simulink model "regcontrol_model"  (Simulink 9.1)
settings: Solver=VariableStepAuto  StartTime=0.0  StopTime=10.0  RelTol=1e-3
values from neighbouring files (symbols this model uses):
  BandWidth = Simulink.Parameter    [start.m]
  BaseVoltage = Simulink.Parameter    [start.m]
  CogenEnabled = false    [regcontrol_emulator.m]    (also in start.m = Simulink.Parameter)
  IsReversible = Simulink.Parameter    [start.m]
  LDC_Z = Simulink.Parameter    [start.m]
  PTratio = Simulink.Parameter    [start.m]
  RevBand = Simulink.Parameter    [start.m]
  RevVreg = Simulink.Parameter    [start.m]
  TapLimitPerChange = Simulink.Parameter    [start.m]
  UsingRegulatedBus = Simulink.Parameter    [start.m]
  Vlimit = Simulink.Parameter    [start.m]
  Vreg = Simulink.Parameter    [start.m]
undefined symbols (not defined in the file or in its folder): ControlModes, m, n
libraries: simulink x3
(part 2 of 2)

== stateflow chart Queue Handler ==
  settings: enableNonTerminalStates=1
  state Executive [parallel]
    settings: executionOrder=1
    state Asleep
      ex: Status.data = Statuses.READY; % reset status
      INTERNAL_DONE = false;
      EXECUTIVE_DONE = false;
    state DoNearestActions
      state WaitOnPeek
        en: send(QUEUE_PEEK, Internal);
      state WaitOnPop
        en: send(QUEUE_POP, Internal);
      state ErrorNoItems
        en: Status.data = ...
        Statuses.ERROR;
        send(Status);
      (default) -> (junction 902) : % do only those actions with the same delay time as the first action time return time
          | {q_len_initial = GetQueueSize;
          | PendingActionsCompleted = false; % local for now
          | }
      (junction 902) -> (junction 903) [order 1] : [q_len_initial > 0]
      (junction 902) -> Executive.DoNearestActions.ErrorNoItems [order 2]
      (junction 903) -> WaitOnPeek : {INTERNAL_DONE = false;
          | ActionTime = ExternalAT; % peek with given AT
          | }
      (junction 905) -> (junction 904) [order 1] : [jj <= q_len_initial]
      (junction 904) -> Executive.DoNearestActions.WaitOnPop : {INTERNAL_DONE = false;}
      WaitOnPeek -> (junction 905) : [INTERNAL_DONE]
          | {ActionTime = Out(QF.Time);
          | QHour = Out(QF.Hour);
          | QSec = Out(QF.Sec);
          | jj = 1;}
      Executive.DoNearestActions.WaitOnPop -> (junction 906) : [INTERNAL_DONE]
          | %send(DoPendingAction);
      (junction 906) -> (junction 905) : {jj = jj + 1;}
      (junction 905) -> (junction 908) [order 2]
      Executive.DoNearestActions.ErrorNoItems -> (junction 907)
      (junction 908) -> (junction 907)
      (junction 907) -> (junction 909) : {EXECUTIVE_DONE = true;}
    state DoAllActions
      state WaitOnPop
        en: send(QUEUE_POP, Internal);
      state ErrorNoItems
        en: Status.data = ...
        Statuses.ERROR;
        send(Status);
      (default) -> (junction 923) : {q_len_initial = GetQueueSize;}
      (junction 923) -> (junction 924) [order 1] : [q_len_initial ~= 0]
      (junction 923) -> Executive.DoAllActions.ErrorNoItems [order 2]
      (junction 924) -> (junction 926) : {ActionTime = ExternalAT;
          | jj = 1;}
      (junction 926) -> (junction 925) [order 1] : [jj <= q_len_initial]
      (junction 925) -> Executive.DoAllActions.WaitOnPop : {INTERNAL_DONE = false;}
      (junction 927) -> (junction 926) : {jj = jj + 1;}
      (junction 926) -> (junction 929) [order 2]
      Executive.DoAllActions.WaitOnPop -> (junction 927) : [INTERNAL_DONE]
          | %send(DoPendingAction);
      Executive.DoAllActions.ErrorNoItems -> (junction 928)
      (junction 929) -> (junction 928)
      (junction 928) -> (junction 930) : {EXECUTIVE_DONE = true;}
    state Pushing
      en: send(QUEUE_PUSH, Internal);
    state DeletingByHandle
      en: send(QUEUE_DELETE, Internal);
    state Peeking
      en: send(QUEUE_PEEK, Internal);
    state Popping
      en: send(QUEUE_POP, Internal);
    state ReadyAgain
      Status.data = Statuses.READY;
      send(Status);
    Executive.Asleep -> Executive.DeletingByHandle [order 6] : QueueAction[QueueAction.data == ...
        | QueueActions.DELETE]
    Executive.Asleep -> Executive.Peeking [order 5] : QueueAction[QueueAction.data == ...
        | QueueActions.PEEK]
    Executive.Asleep -> Executive.Popping [order 4] : QueueAction[QueueAction.data == ...
        | QueueActions.POP]
    (default) -> Executive.Asleep
    Executive.Asleep -> Executive.Pushing [order 3] : QueueAction[QueueAction.data == ...
        | QueueActions.PUSH]
    Executive.Asleep -> DoAllActions [order 2] : QueueAction[QueueAction.data == ...
        | QueueActions.DO_ALL_ACTIONS]
    ReadyAgain -> Executive.Asleep
    Executive.Asleep -> DoNearestActions [order 1] : QueueAction[QueueAction.data == DO_NEAREST_ACTIONS]
    Executive.Pushing -> ReadyAgain : [INTERNAL_DONE]
    Executive.Popping -> ReadyAgain : [INTERNAL_DONE]
    Executive.DeletingByHandle -> ReadyAgain : [INTERNAL_DONE]
    Executive.Peeking -> ReadyAgain : [INTERNAL_DONE]
    DoAllActions -> ReadyAgain : [EXECUTIVE_DONE]
    DoNearestActions -> ReadyAgain : [EXECUTIVE_DONE]
  state Internal [parallel]
    settings: executionOrder=2
    state Asleep
    state Popping
      (default) -> (junction 955) : % delete from beginning, t<= ActionTime:
          | {q_len = GetQueueSize;
          | ii = 1;
          | }
      (junction 955) -> (junction 952) [order 1] : [ii <= q_len]
      (junction 952) -> (junction 953)
      (junction 953) -> (junction 954) [order 1] : [GetElemTime(ii) <= ActionTime]
      (junction 953) -> (junction 956) [order 2]
      (junction 954) -> (junction 958) : {Out = GetElem(ii);
          | ReduceQueue(ii);
          | send(DoPendingAction);}
          | % break
      (junction 956) -> (junction 955) : {ii = ii + 1;}
      (junction 955) -> (junction 957) [order 2]
      (junction 958) -> (junction 957)
      (junction 957) -> (junction 959)
      (junction 959) -> (junction 960) [order 1] : [QueueEmpty.data == true]
      (junction 959) -> (junction 961) [order 2]
      (junction 960) -> (junction 962) : {send(QueueEmpty);}
      (junction 962) -> (junction 961)
      (junction 961) -> (junction 963) : {INTERNAL_DONE = true;}
    state DeletingByHandle
      (default) -> (junction 982) : % delete from beginning, t<= ActionTime:
          | {q_len = GetQueueSize;
          | ii = 1;
          | }
      (junction 982) -> (junction 979) [order 1] : [ii <= q_len]
      (junction 979) -> (junction 980)
      (junction 980) -> (junction 981) [order 1] : [GetElemHandle(ii) == ExternalHandle]
      (junction 980) -> (junction 983) [order 2]
      (junction 981) -> (junction 985) : {Out = GetElem(ii);
          | ReduceQueue(ii);}
          | % break
      (junction 983) -> (junction 982) : {ii = ii + 1;}
      (junction 982) -> (junction 984) [order 2]
      (junction 985) -> (junction 984)
      (junction 984) -> (junction 986)
      (junction 986) -> (junction 987) [order 1] : [QueueEmpty.data == true]
      (junction 986) -> (junction 988) [order 2]
      (junction 987) -> (junction 989) : {send(QueueEmpty);}
      (junction 989) -> (junction 988)
      (junction 988) -> (junction 990) : {INTERNAL_DONE = true;}
    state Pushing
      (default) -> (junction 1009) : % insert into queue right before item of greater or equal execution time
          | {q_cand = In'; % transposition to 1 x 5
          | q_len = GetQueueSize; %size(queue, 3);
          | ii = 1;
          | }
      (junction 1009) -> (junction 1006) [order 1] : [ii <= q_len]
      (junction 1006) -> (junction 1007)
      (junction 1007) -> (junction 1008) [order 1] : [q_cand(1,QF.Time) <= GetElemTime(ii)]
      (junction 1007) -> (junction 1010) [order 2]
      (junction 1008) -> (junction 1012) : {
          | ExpandQueue(ii);}
          | % break
      (junction 1010) -> (junction 1009) : {ii = ii + 1;}
      (junction 1009) -> (junction 1011) [order 2] : {ExpandQueue(q_len+1);}
      (junction 1012) -> (junction 1011)
      (junction 1011) -> (junction 1013) : %{send(DONE_PUSHING, Executive.Pushing);}
          | {INTERNAL_DONE = true;}
    state Peeking
      (default) -> (junction 1027) : % pop without deletion
          | {q_len = GetQueueSize;
          | ii = 1;
          | }
      (junction 1027) -> (junction 1024) [order 1] : [ii <= q_len]
      (junction 1024) -> (junction 1025)
      (junction 1025) -> (junction 1026) [order 1] : [GetElemTime(ii) <= ActionTime]
      (junction 1025) -> (junction 1028) [order 2]
      (junction 1026) -> (junction 1030) : {Out = GetElem(ii);}
          | % break
      (junction 1028) -> (junction 1027) : {ii = ii + 1;}
      (junction 1027) -> (junction 1029) [order 2]
      (junction 1030) -> (junction 1029)
      (junction 1029) -> (junction 1031) : {INTERNAL_DONE = true;}
    (default) -> Internal.Asleep
    Internal.Asleep -> Internal.Pushing [order 1] : QUEUE_PUSH
    Internal.Pushing -> Internal.Asleep : [INTERNAL_DONE]
    Internal.Asleep -> Internal.Popping [order 2] : QUEUE_POP
    Internal.Popping -> Internal.Asleep : [INTERNAL_DONE]
    Internal.Asleep -> Internal.Peeking [order 3] : QUEUE_PEEK
    Internal.Peeking -> Internal.Asleep : [INTERNAL_DONE]
    Internal.Asleep -> Internal.DeletingByHandle [order 4] : QUEUE_DELETE
    Internal.DeletingByHandle -> Internal.Asleep : [INTERNAL_DONE]
  state QF % Queue Fields [group]
  data: Handle local double =1; Time local double =2; Hour local double =3; Sec local double =4; ActionCode local double =5; depth function_input double; h function_output double; qs function_output double; depth function_input double; et function_output double; elem function_output double; depth function_input double; depth function_input double; depth function_input double; DoPendingAction output boolean =true; QueueAction input Enum: QueueActions; Status output Enum: Statuses; Out output double size=[1 5]; queue output double size=[1 5 50]; q_len local double =0; PendingActionsCompleted local boolean =false; QHour local double; QSec local double; q_cand local double size=[1 5]; In input double size=5; qwriteflag local boolean =false; ii local uint8; jj local uint8; q_len_initial local double; EXECUTIVE_DONE local boolean =false; INTERNAL_DONE local boolean =false;; ExternalAT input double =100; ActionTime local double; QueueEmpty output boolean =false; ExternalHandle input uint8
  events: QUEUE_POP local FUNCTION_CALL_EVENT; QUEUE_PUSH local FUNCTION_CALL_EVENT; QUEUE_PEEK local FUNCTION_CALL_EVENT; QUEUE_DELETE local FUNCTION_CALL_EVENT
  function h = GetElemHandle(depth):
    | function h = GetElemHandle(depth)
    |     h = zeros(1,1);
    |     if ~isempty(queue)
    |         h = queue(1,QF.Handle,ii);
    |         h = cast(h, 'uint8'); % for comparison with ExternalHandle
    |     else
    | end
  function qs = GetQueueSize:
    | function qs = GetQueueSize
    | %     coder.extrinsic('exist');
    | %     eq = zeros(1,1,'double');
    | %     eq = exist('queue');
    | %     if eq == 1 && ~isempty(queue)
    | %         qs = size(queue, 3);
    | %     else % eq ~= 1 || size == 0
    | %         qs = 0;
    | %     end
    |     if ~qwriteflag % can't read intial value of empty queue, so depend on flag
    |         queue = zeros(1,5);
    |         qs = 0;
    |         QueueEmpty.data = true;
    |         qwriteflag = true;
    |     elseif isequal(queue,zeros(1,5)) % case of empty queue (still 1 element)
    |         qs = 0;
    |         QueueEmpty.data = true;
    |     else
    |         qs = size(queue,3);
    |         QueueEmpty.data = false;
    |     end
    | end
  function et = GetElemTime(depth):
    | function et = GetElemTime(depth)
    |     et = zeros(1,1);
    |     if ~isempty(queue)
    |         et = queue(1,QF.Time,ii);
    |     else
    |     end
    | end
  function elem = GetElem(depth):
    | function elem = GetElem(depth)
    |     elem = zeros(1,5);
    |     elem(1,:) = queue(:,:,depth);
    | end
  function ExpandQueue(depth):
    | function ExpandQueue(depth)
    |     rhs = queue(:,:,depth:q_len); % the RHS of the queue
    |     bigger = zeros(1,5,q_len+1);
    |     bigger(:,:,1:(depth-1)) = queue(:,:,1:(depth-1)); % copy LHS
    |     bigger(:,:,depth) = q_cand; % inserting element at end of LHS
    |     %queue(:,:,depth) = q_cand; 
    |     bigger(:,:, (depth+1):(q_len+1)) = rhs; % tack on RHS again
    |     queue = bigger;
    | end
  function ReduceQueue(depth):
    | function ReduceQueue(depth)
    |     rhs = queue(:,:,(depth+1):q_len); % excluding element at depth
    |     smaller = zeros(1,5,q_len-1);
    |     smaller(:,:,1:(depth-1)) = queue(:,:,1:(depth-1)); % lhs, excl. depth
    |     smaller(:,:,depth:(q_len-1)) = rhs; % tack on rhs
    |     queue = smaller;
    | end
